simulink model "test_adc_clip"  (Simulink 7.0)
settings: Solver=ode45  StartTime=0.0  StopTime=10.0  RelTol=1e-3
libraries: xbsIndex_r4 x31, xps_library x1
settings Model: Creator=dsp  LastModifiedBy=dsp

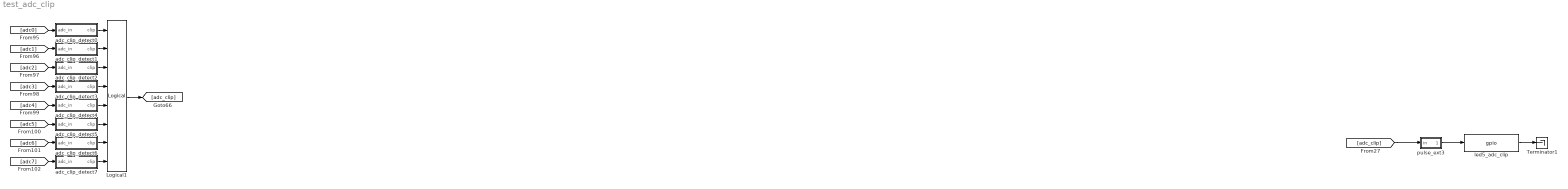
== system test_adc_clip ==
  Logical1 : xbsIndex_r4/Logical  logical_function=OR  inputs=8  en=off  latency=1  precision=Full  arith_type=Unsigned  n_bits=8  bin_pt=2  align_bp=on  dbl_ovrd=off  block_type=logical
      settings: xl_area=[0, 0, 0, 0, 0, 0, 0]
  Terminator1 : Terminator
  adc_clip_detect0 : Subsystem  mask{n_bits=8}
      mask prompts: n_bits "Number of ADC bits"
  adc_clip_detect1 : Subsystem  mask{n_bits=8}
      mask prompts: n_bits "Number of ADC bits"
  adc_clip_detect2 : Subsystem  mask{n_bits=8}
      mask prompts: n_bits "Number of ADC bits"
  adc_clip_detect3 : Subsystem  mask{n_bits=8}
      mask prompts: n_bits "Number of ADC bits"
  adc_clip_detect4 : Subsystem  mask{n_bits=8}
      mask prompts: n_bits "Number of ADC bits"
  adc_clip_detect5 : Subsystem  mask{n_bits=8}
      mask prompts: n_bits "Number of ADC bits"
  adc_clip_detect6 : Subsystem  mask{n_bits=8}
      mask prompts: n_bits "Number of ADC bits"
  adc_clip_detect7 : Subsystem  mask{n_bits=8}
      mask prompts: n_bits "Number of ADC bits"
  led5_adc_clip : xps_library/gpio  Tag=xps:gpio  SystemSampleTime=-1  io_group=iBOB:led  io_dir=out  arith_type=Boolean  bitwidth=1  bin_pt=0  bit_index=5  sample_period=1  use_single_ended=off  use_ddr=off  reg_iob=on  reg_clk_phase=0  termination=None
      link override convert: arith_type=Boolean  n_bits=1  bin_pt=0
  pulse_ext3 : Subsystem  mask{pulse_len=2^23}
      mask prompts: pulse_len "Length of Pulse"
      mask init:
      | bits = ceil(log2(pulse_len+1));
  wires:
  [adc0] -> adc_clip_detect0/1(adc_in)
  [adc1] -> adc_clip_detect1/1(adc_in)
  [adc2] -> adc_clip_detect2/1(adc_in)
  [adc3] -> adc_clip_detect3/1(adc_in)
  [adc4] -> adc_clip_detect4/1(adc_in)
  [adc5] -> adc_clip_detect5/1(adc_in)
  [adc6] -> adc_clip_detect6/1(adc_in)
  [adc7] -> adc_clip_detect7/1(adc_in)
  adc_clip_detect0/1(clip) -> Logical1/1
  adc_clip_detect1/1(clip) -> Logical1/2
  adc_clip_detect2/1(clip) -> Logical1/3
  adc_clip_detect3/1(clip) -> Logical1/4
  adc_clip_detect4/1(clip) -> Logical1/5
  adc_clip_detect5/1(clip) -> Logical1/6
  adc_clip_detect6/1(clip) -> Logical1/7
  adc_clip_detect7/1(clip) -> Logical1/8
  Logical1/1 -> [adc_clip]
  [adc_clip] -> pulse_ext3/1(in)
  pulse_ext3/1(out) -> led5_adc_clip/1
  led5_adc_clip/1 -> Terminator1/1

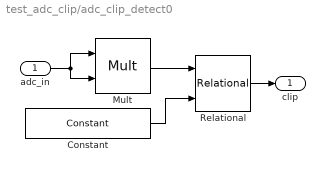
== system test_adc_clip/adc_clip_detect0 ==
  adc_in : Inport
  Constant : xbsIndex_r4/Constant  arith_type=Unsigned  const=((2^(n_bits-1)-1)/(2^(n_bits-1)))^2  n_bits=2*n_bits +1  bin_pt=n_bits*2  explicit_period=on  period=1  equ=P=C  opselect=C  inp2=PCIN>>17  opr=+  inp1=P  carry=CIN  dbl_ovrd=off  block_type=constant
  Mult : xbsIndex_r4/Mult  precision=Full  arith_type="Signed  (2's comp)"  n_bits=16  bin_pt=14  quantization=Truncate  overflow=Wrap  en=off  latency=3  dbl_ovrd=off  use_behavioral_HDL=off  use_embedded=on  opt=Speed  optimum_pipeline=on  pipeline=on  use_rpm=on  placement_style=Triangular  block_type=mult
      settings: infoedit=Hardware notes: To use the internal pipeline stage of the dedicated multiplier you must select 'Pipeline for maximum performance'.  block_version=10.1.3
  Relational : xbsIndex_r4/Relational  mode=a>=b  en=off  latency=1  dbl_ovrd=off  block_type=relational
      settings: block_version=10.1.3
  clip : Outport
  wires:
  adc_in/1 -> Mult/2, Mult/1
  Mult/1 -> Relational/1
  Constant/1 -> Relational/2
  Relational/1 -> clip/1

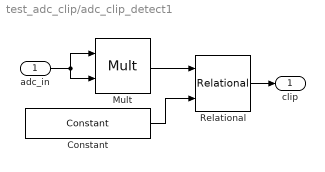
== system test_adc_clip/adc_clip_detect1 ==
  adc_in : Inport
  Constant : xbsIndex_r4/Constant  arith_type=Unsigned  const=((2^(n_bits-1)-1)/(2^(n_bits-1)))^2  n_bits=2*n_bits +1  bin_pt=n_bits*2  explicit_period=on  period=1  equ=P=C  opselect=C  inp2=PCIN>>17  opr=+  inp1=P  carry=CIN  dbl_ovrd=off  block_type=constant
  Mult : xbsIndex_r4/Mult  precision=Full  arith_type="Signed  (2's comp)"  n_bits=16  bin_pt=14  quantization=Truncate  overflow=Wrap  en=off  latency=3  dbl_ovrd=off  use_behavioral_HDL=off  use_embedded=on  opt=Speed  optimum_pipeline=on  pipeline=on  use_rpm=on  placement_style=Triangular  block_type=mult
      settings: infoedit=Hardware notes: To use the internal pipeline stage of the dedicated multiplier you must select 'Pipeline for maximum performance'.  block_version=10.1.3
  Relational : xbsIndex_r4/Relational  mode=a>=b  en=off  latency=1  dbl_ovrd=off  block_type=relational
      settings: block_version=10.1.3
  clip : Outport
  wires:
  Relational/1 -> clip/1
  Constant/1 -> Relational/2
  Mult/1 -> Relational/1
  adc_in/1 -> Mult/1, Mult/2

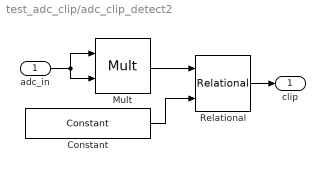
== system test_adc_clip/adc_clip_detect2 ==
  adc_in : Inport
  Constant : xbsIndex_r4/Constant  arith_type=Unsigned  const=((2^(n_bits-1)-1)/(2^(n_bits-1)))^2  n_bits=2*n_bits +1  bin_pt=n_bits*2  explicit_period=on  period=1  equ=P=C  opselect=C  inp2=PCIN>>17  opr=+  inp1=P  carry=CIN  dbl_ovrd=off  block_type=constant
  Mult : xbsIndex_r4/Mult  precision=Full  arith_type="Signed  (2's comp)"  n_bits=16  bin_pt=14  quantization=Truncate  overflow=Wrap  en=off  latency=3  dbl_ovrd=off  use_behavioral_HDL=off  use_embedded=on  opt=Speed  optimum_pipeline=on  pipeline=on  use_rpm=on  placement_style=Triangular  block_type=mult
      settings: infoedit=Hardware notes: To use the internal pipeline stage of the dedicated multiplier you must select 'Pipeline for maximum performance'.  block_version=10.1.3
  Relational : xbsIndex_r4/Relational  mode=a>=b  en=off  latency=1  dbl_ovrd=off  block_type=relational
      settings: block_version=10.1.3
  clip : Outport
  wires:
  adc_in/1 -> Mult/2, Mult/1
  Mult/1 -> Relational/1
  Constant/1 -> Relational/2
  Relational/1 -> clip/1

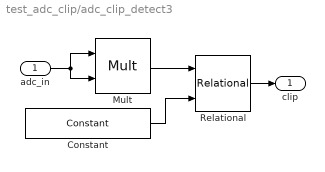
== system test_adc_clip/adc_clip_detect3 ==
  adc_in : Inport
  Constant : xbsIndex_r4/Constant  arith_type=Unsigned  const=((2^(n_bits-1)-1)/(2^(n_bits-1)))^2  n_bits=2*n_bits +1  bin_pt=n_bits*2  explicit_period=on  period=1  equ=P=C  opselect=C  inp2=PCIN>>17  opr=+  inp1=P  carry=CIN  dbl_ovrd=off  block_type=constant
  Mult : xbsIndex_r4/Mult  precision=Full  arith_type="Signed  (2's comp)"  n_bits=16  bin_pt=14  quantization=Truncate  overflow=Wrap  en=off  latency=3  dbl_ovrd=off  use_behavioral_HDL=off  use_embedded=on  opt=Speed  optimum_pipeline=on  pipeline=on  use_rpm=on  placement_style=Triangular  block_type=mult
      settings: infoedit=Hardware notes: To use the internal pipeline stage of the dedicated multiplier you must select 'Pipeline for maximum performance'.  block_version=10.1.3
  Relational : xbsIndex_r4/Relational  mode=a>=b  en=off  latency=1  dbl_ovrd=off  block_type=relational
      settings: block_version=10.1.3
  clip : Outport
  wires:
  Relational/1 -> clip/1
  Constant/1 -> Relational/2
  Mult/1 -> Relational/1
  adc_in/1 -> Mult/1, Mult/2

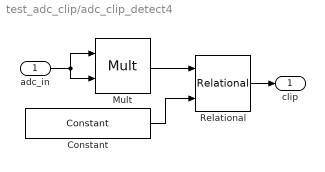
== system test_adc_clip/adc_clip_detect4 ==
  adc_in : Inport
  Constant : xbsIndex_r4/Constant  arith_type=Unsigned  const=((2^(n_bits-1)-1)/(2^(n_bits-1)))^2  n_bits=2*n_bits +1  bin_pt=n_bits*2  explicit_period=on  period=1  equ=P=C  opselect=C  inp2=PCIN>>17  opr=+  inp1=P  carry=CIN  dbl_ovrd=off  block_type=constant
  Mult : xbsIndex_r4/Mult  precision=Full  arith_type="Signed  (2's comp)"  n_bits=16  bin_pt=14  quantization=Truncate  overflow=Wrap  en=off  latency=3  dbl_ovrd=off  use_behavioral_HDL=off  use_embedded=on  opt=Speed  optimum_pipeline=on  pipeline=on  use_rpm=on  placement_style=Triangular  block_type=mult
      settings: infoedit=Hardware notes: To use the internal pipeline stage of the dedicated multiplier you must select 'Pipeline for maximum performance'.  block_version=10.1.3
  Relational : xbsIndex_r4/Relational  mode=a>=b  en=off  latency=1  dbl_ovrd=off  block_type=relational
      settings: block_version=10.1.3
  clip : Outport
  wires:
  Relational/1 -> clip/1
  Constant/1 -> Relational/2
  Mult/1 -> Relational/1
  adc_in/1 -> Mult/1, Mult/2

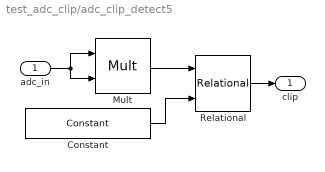
== system test_adc_clip/adc_clip_detect5 ==
  adc_in : Inport
  Constant : xbsIndex_r4/Constant  arith_type=Unsigned  const=((2^(n_bits-1)-1)/(2^(n_bits-1)))^2  n_bits=2*n_bits +1  bin_pt=n_bits*2  explicit_period=on  period=1  equ=P=C  opselect=C  inp2=PCIN>>17  opr=+  inp1=P  carry=CIN  dbl_ovrd=off  block_type=constant
  Mult : xbsIndex_r4/Mult  precision=Full  arith_type="Signed  (2's comp)"  n_bits=16  bin_pt=14  quantization=Truncate  overflow=Wrap  en=off  latency=3  dbl_ovrd=off  use_behavioral_HDL=off  use_embedded=on  opt=Speed  optimum_pipeline=on  pipeline=on  use_rpm=on  placement_style=Triangular  block_type=mult
      settings: infoedit=Hardware notes: To use the internal pipeline stage of the dedicated multiplier you must select 'Pipeline for maximum performance'.  block_version=10.1.3
  Relational : xbsIndex_r4/Relational  mode=a>=b  en=off  latency=1  dbl_ovrd=off  block_type=relational
      settings: block_version=10.1.3
  clip : Outport
  wires:
  adc_in/1 -> Mult/2, Mult/1
  Mult/1 -> Relational/1
  Constant/1 -> Relational/2
  Relational/1 -> clip/1

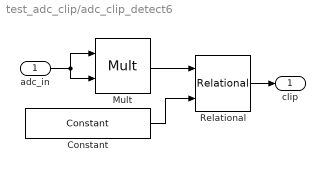
== system test_adc_clip/adc_clip_detect6 ==
  adc_in : Inport
  Constant : xbsIndex_r4/Constant  arith_type=Unsigned  const=((2^(n_bits-1)-1)/(2^(n_bits-1)))^2  n_bits=2*n_bits +1  bin_pt=n_bits*2  explicit_period=on  period=1  equ=P=C  opselect=C  inp2=PCIN>>17  opr=+  inp1=P  carry=CIN  dbl_ovrd=off  block_type=constant
  Mult : xbsIndex_r4/Mult  precision=Full  arith_type="Signed  (2's comp)"  n_bits=16  bin_pt=14  quantization=Truncate  overflow=Wrap  en=off  latency=3  dbl_ovrd=off  use_behavioral_HDL=off  use_embedded=on  opt=Speed  optimum_pipeline=on  pipeline=on  use_rpm=on  placement_style=Triangular  block_type=mult
      settings: infoedit=Hardware notes: To use the internal pipeline stage of the dedicated multiplier you must select 'Pipeline for maximum performance'.  block_version=10.1.3
  Relational : xbsIndex_r4/Relational  mode=a>=b  en=off  latency=1  dbl_ovrd=off  block_type=relational
      settings: block_version=10.1.3
  clip : Outport
  wires:
  Relational/1 -> clip/1
  Constant/1 -> Relational/2
  Mult/1 -> Relational/1
  adc_in/1 -> Mult/1, Mult/2

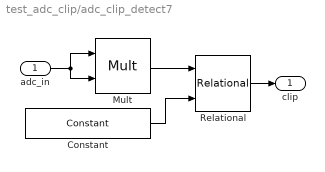
== system test_adc_clip/adc_clip_detect7 ==
  adc_in : Inport
  Constant : xbsIndex_r4/Constant  arith_type=Unsigned  const=((2^(n_bits-1)-1)/(2^(n_bits-1)))^2  n_bits=2*n_bits +1  bin_pt=n_bits*2  explicit_period=on  period=1  equ=P=C  opselect=C  inp2=PCIN>>17  opr=+  inp1=P  carry=CIN  dbl_ovrd=off  block_type=constant
  Mult : xbsIndex_r4/Mult  precision=Full  arith_type="Signed  (2's comp)"  n_bits=16  bin_pt=14  quantization=Truncate  overflow=Wrap  en=off  latency=3  dbl_ovrd=off  use_behavioral_HDL=off  use_embedded=on  opt=Speed  optimum_pipeline=on  pipeline=on  use_rpm=on  placement_style=Triangular  block_type=mult
      settings: infoedit=Hardware notes: To use the internal pipeline stage of the dedicated multiplier you must select 'Pipeline for maximum performance'.  block_version=10.1.3
  Relational : xbsIndex_r4/Relational  mode=a>=b  en=off  latency=1  dbl_ovrd=off  block_type=relational
      settings: block_version=10.1.3
  clip : Outport
  wires:
  adc_in/1 -> Mult/2, Mult/1
  Mult/1 -> Relational/1
  Constant/1 -> Relational/2
  Relational/1 -> clip/1

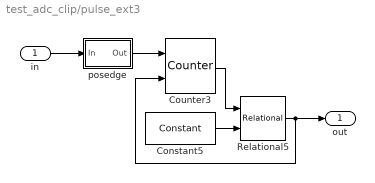
== system test_adc_clip/pulse_ext3 ==
  in : Inport  OutDataType=sfix(16)  OutScaling=2^0
  Constant5 : xbsIndex_r4/Constant  arith_type=Unsigned  const=pulse_len  n_bits=bits  bin_pt=0  explicit_period=off  period=1  equ=P=C  opselect=C  inp2=PCIN>>17  opr=+  inp1=P  carry=CIN  dbl_ovrd=off  block_type=constant
  Counter3 : xbsIndex_r4/Counter  cnt_type=Free Running  cnt_to=1023  operation=Up  start_count=0  cnt_by_val=1  arith_type=Unsigned  n_bits=bits  bin_pt=0  load_pin=off  rst=on  en=on  explicit_period=on  period=1  dbl_ovrd=off  use_behavioral_HDL=off  use_rpm=on  implementation=Fabric  block_type=counter
      settings: xl_area=[0, 0, 0, 0, 0, 0, 0]
  Relational5 : xbsIndex_r4/Relational  mode=a!=b  en=off  latency=0  dbl_ovrd=off  block_type=relational
      settings: xl_area=[0, 0, 0, 0, 0, 0, 0]  block_version=10.1.3
  posedge : Subsystem  Tag=Rising Edge Detector
  out : Outport  OutDataType=sfix(16)  OutScaling=2^0
  wires:
  Counter3/1 -> Relational5/1
  Constant5/1 -> Relational5/2
  Relational5/1 -> Counter3/2, out/1
  in/1 -> posedge/1(In)
  posedge/1(Out) -> Counter3/1

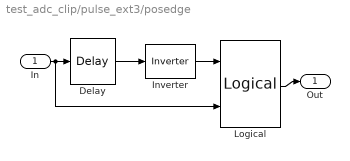
== system test_adc_clip/pulse_ext3/posedge ==
  In : Inport  OutDataType=sfix(16)  OutScaling=2^0
  Delay : xbsIndex_r4/Delay  en=off  latency=1  dbl_ovrd=off  reg_retiming=off  block_type=delay
      settings: xl_area=[0, 0, 0, 0, 0, 0, 0]
  Inverter : xbsIndex_r4/Inverter  en=off  latency=0  dbl_ovrd=off  block_type=inv
      settings: xl_area=[0, 0, 0, 0, 0, 0, 0]
  Logical : xbsIndex_r4/Logical  logical_function=AND  inputs=2  en=off  latency=0  precision=Full  arith_type=Unsigned  n_bits=8  bin_pt=2  align_bp=on  dbl_ovrd=off  block_type=logical
      settings: xl_area=[0, 0, 0, 0, 0, 0, 0]
  Out : Outport  OutDataType=sfix(16)  OutScaling=2^0
  wires:
  Delay/1 -> Inverter/1
  Inverter/1 -> Logical/1
  In/1 -> Delay/1, Logical/2
  Logical/1 -> Out/1
